simulink model "observer_test"  (R2022a)
settings: Solver=FixedStepAuto  StartTime=0.0  StopTime=10.0  FixedStep=Ts  RelTol=1e-3
values from neighbouring files (symbols this model uses):
  A = A(1:2,1:2)    [observer_design.m]
  Aobs = A-L*C    [observer_design.m]
  B = B(1:2,1)    [observer_design.m]
  Bobs = [B L]    [observer_design.m]
  C = C(1,1:2)    [observer_design.m]
  Cobs = eye(2)    [observer_design.m]
  Dobs = [0,0 ... (first row only)    [observer_design.m]
  K = -acker(A,B,poles)    [observer_design.m]
  ss_d = c2d(ss_c,Ts,'zoh')    [observer_design.m]
undefined symbols (not defined in the file or in its folder): Discrete, Time
libraries: ctrlSharedLib x1
settings Model: Creator=michi  LastModifiedBy=michi

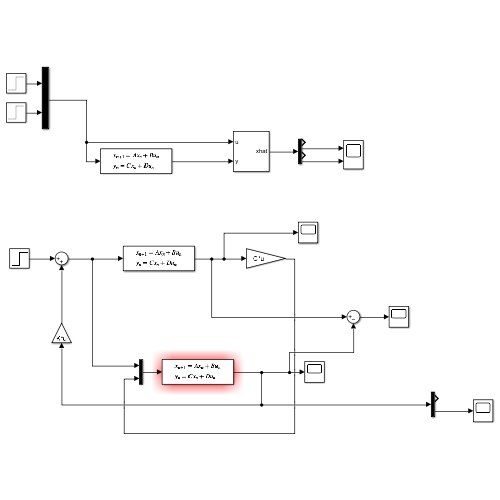
[thumbnail: Simulink's stored preview of the top-level diagram]
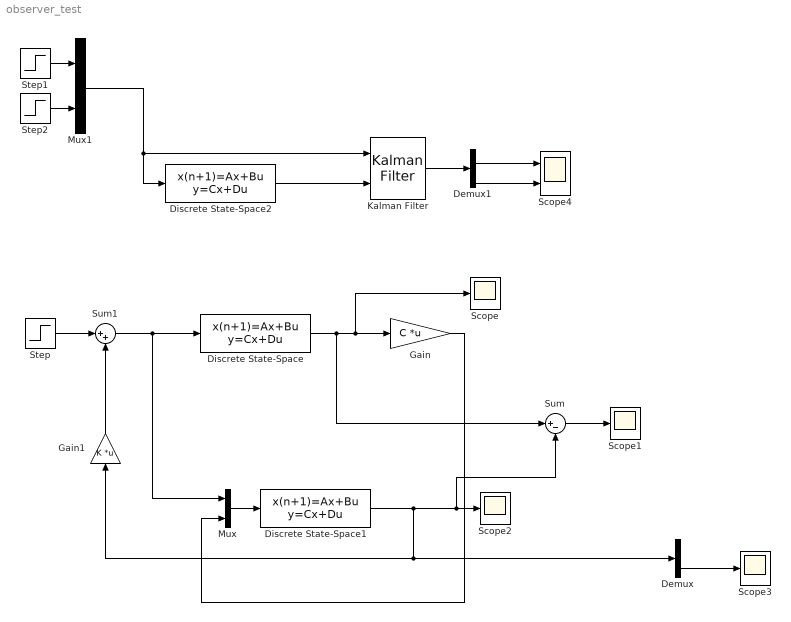
== system observer_test ==
  Demux : Demux  Outputs=2
  Demux1 : Demux
  Discrete State-Space : DiscreteStateSpace  A=A  B=B  C=eye(2)  D=[0;0]  InitialCondition=[10 -10]'  SampleTime=-1
  Discrete State-Space1 : DiscreteStateSpace  A=Aobs  B=Bobs  C=Cobs  D=Dobs  InitialCondition=[0,0]  SampleTime=-1
  Discrete State-Space2 : DiscreteStateSpace  A=ss_d.A  B=ss_d.B  C=ss_d.C  D=ss_d.D  InitialCondition=[10 -10 10 -10]'  SampleTime=-1
  Gain : Gain  Gain=C  Multiplication=Matrix(K*u)
  Gain1 : Gain  Gain=K  Multiplication=Matrix(K*u)
  Kalman Filter : ctrlSharedLib/Kalman Filter  TimeDomain=Discrete-Time  UseCurrentEstimator=on  ModelSource=Individual A, B, C, D matrices  ModelSourceVariable=ss(0.95,1,1,0,1)  A=ss_d.A  B=ss_d.B  C=ss_d.C  D=ss_d.D  NumberOfStates=1  NumberOfInputs=1  NumberOfOutputs=1  InitialEstimateSource=Dialog  X0=0  P0=10  UseK=off  UseGH=off  NumberOfProcessNoiseInputs=1  G=1  TimeInvariantG=on  H=0  TimeInvariantH=on  Q=0.05  TimeInvariantQ=on  R=1  TimeInvariantR=on  N=0  TimeInvariantN=on  AddInputPort=on  AddEnablePort=off  OutputEstimatedY=off  OutputP=off  Ts=-1
  Mux : Mux  Inputs=2
  Mux1 : Mux  Inputs=2
  Scope{,1..3} (4 alike) : Scope
  Scope4 : Scope  NumInputPorts=2
  Step : Step  SampleTime=0
  Step1 : Step  SampleTime=0.035
  Step2 : Step  SampleTime=0.035
  Sum : Sum  Inputs=|+-
  Sum1 : Sum  Inputs=|++
  wires:
  Discrete State-Space/1 -> Sum/1, Scope/1, Gain/1
  Step/1 -> Sum1/1
  Discrete State-Space1/1 -> Gain1/1, Demux/1, Sum/2, Scope2/1
  Gain1/1 -> Sum1/2
  Sum/1 -> Scope1/1
  Sum1/1 -> Discrete State-Space/1, Mux/1
  Mux/1 -> Discrete State-Space1/1
  Gain/1 -> Mux/2
  Demux/2 -> Scope3/1
  Discrete State-Space2/1 -> Kalman Filter/2
  Step1/1 -> Mux1/1
  Step2/1 -> Mux1/2
  Mux1/1 -> Kalman Filter/1, Discrete State-Space2/1
  Kalman Filter/1 -> Demux1/1
  Demux1/2 -> Scope4/1
  Demux1/4 -> Scope4/2
